simulink model "Control_v2"  (R2019b)
settings: Solver=FixedStepAuto  StartTime=0.0  StopTime=10  FixedStep=str2num(Step_size)  RelTol=1e-3
model workspace: external: MATLAB File H:\4-project\matlab\github\Sim-v2\bicopter_sim\Bicopter_DataFile14.m (data not in the file)
values from neighbouring files (symbols this model uses):
  b = [5,1,5,4]    [init_ADRC_val.m]    (also in init_Non_Linear_ADRC_val.m = 0.5*[1,    1, 6,  6]')
  b_sep = gains(5:8)    [get_ADRC_parameters.m]    (also in get_adrc_sep.m = [  2   7    6   7]; get_adrc_sep_kalman.m = [  2   2    6   7])
  C = [eye(4),zeros(4,8)]    [init_ADRC_val.m]
  C_air = 0.0025    [Sim_Script.m]
  d_f_phi = 100    [Sim_Script.m]
  d_f_psi = 25    [Sim_Script.m]
  d_f_theta = 10    [Sim_Script.m]
  d_f_z = 100    [Sim_Script.m]
  eps_sep = 0.7*[1 1 1 1]    [get_ADRC_parameters.m]    (also in get_adrc_sep.m = [0.7 0.3 0.3 0.35]; get_adrc_sep_kalman.m = [0.7 0.7 0.3 0.35])
  epsi = 1.5    [init_Non_Linear_ADRC_val.m]
  euler_source = 1    [Sim_Script.m]
  freq_cut_angvel_phi = 75    [Sim_Script.m]
  freq_cut_angvel_psi = 75    [Sim_Script.m]
  freq_cut_angvel_theta = 50    [Sim_Script.m]
  g = 9.81    [Sim_Script.m]
  K = place(A1,B1,w00(1:8))    [init_ADRC_val.m]
  L = place(A',C',8*w00)'    [init_ADRC_val.m]
  method = STSC_controller    (= 2)    [Sim_Script.m]
  method_angle_plane_sw = plane_sw    (= 2)    [Sim_Script.m]
  mult_obs = 10    [init_Non_Linear_ADRC_val.m]
  Noise_gain = 1    [Sim_Script.m]
  PID_VAL_SEP = init_pid_val_sep()    [Sim_Script.m]
  polarity = [-1;1;1;1]    [Sim_Script.m]
  r = [10,5,10,10]    [init_Non_Linear_ADRC_val.m]
  S_phi = 0.001    [Sim_Script.m]
  S_psi = S_phi    (= 0.001)    [Sim_Script.m]
  S_theta = S_phi    (= 0.001)    [Sim_Script.m]
  State_step = [Z_step;Phi_step;Theta_step;Psi_step]    [req_response.m]
  Step_size = step_size    [Sim_Script.m]
  STSC_VAL = init_STSC_val()    [Sim_Script.m]
  time_delay = 1e-6    (= 1e-06)    [Sim_Script.m]
  V_phi = 0.01    [Sim_Script.m]
  V_psi = 0.01    [Sim_Script.m]
  V_theta = 0.01    [Sim_Script.m]
  wc_sep = gains(1:4)    [get_ADRC_parameters.m]    (also in get_adrc_sep.m = [ 5.54   9   6    3]; get_adrc_sep_kalman.m = [ 5.54   9   6    3])
  wo_sep = ga*wc_sep    [get_ADRC_parameters.m]    (also in get_adrc_sep.m; get_adrc_sep_kalman.m)
undefined symbols (not defined in the file or in its folder): Continuous, magnitude, NLADRC_VAL, sigbuilder_block, smiData, Time, X, Y, Z
libraries: sm_lib x141, nesl_utility x20, simulink x19, fuzblock x3, sharedtransform x1, ctrlSharedLib x1
(part 7 of 7)

== system Control_v2/System/Controller/NonLinearADRC/controller_phi2/NLSEF/f_nl1 ==
  e : Inport
  Constant2 : Constant
  Divide : Product  Inputs=*/
  Power : Math  Operator=pow  SignedPower=off  SaturateOnIntegerOverflow=on
  Power1 : Math  Operator=pow  SignedPower=off  SaturateOnIntegerOverflow=on
  Product : Product
  Sign1 : Signum
  Subtract : Sum  Inputs=+-
  Switch : Switch  Criteria=u2 > Threshold  Threshold=NLADRC_VAL(ind,2)
  eta : Constant  Value=NLADRC_VAL(ind,2)
  gamma : Constant  Value=NLADRC_VAL(ind,3)
  fnl : Outport
  wires:
  Switch/1 -> fnl/1
  gamma/1 -> Subtract/1, Power/2
  [abs_err] -> Power/1
  Divide/1 -> Switch/3
  Power1/1 -> Divide/2
  Subtract/1 -> Power1/2
  eta/1 -> Power1/1
  [sign_err] -> Product/2
  Power/1 -> Product/1
  Constant2/1 -> Subtract/2
  e/1 -> [err], [abs_err], Sign1/1
  Product/1 -> Switch/1
  [abs_err] -> Switch/2
  Sign1/1 -> [sign_err]
  [err] -> Divide/1

== system Control_v2/System/Controller/NonLinearADRC/controller_phi3/NLSEF/f_nl ==
  e : Inport
  Constant2 : Constant
  Divide : Product  Inputs=*/
  Power : Math  Operator=pow  SignedPower=off  SaturateOnIntegerOverflow=on
  Power1 : Math  Operator=pow  SignedPower=off  SaturateOnIntegerOverflow=on
  Product : Product
  Sign1 : Signum
  Subtract : Sum  Inputs=+-
  Switch : Switch  Criteria=u2 > Threshold  Threshold=NLADRC_VAL(ind,2)
  eta : Constant  Value=NLADRC_VAL(ind,2)
  gamma : Constant  Value=NLADRC_VAL(ind,3)
  fnl : Outport
  wires:
  Switch/1 -> fnl/1
  gamma/1 -> Subtract/1, Power/2
  [abs_err] -> Power/1
  Divide/1 -> Switch/3
  Power1/1 -> Divide/2
  Subtract/1 -> Power1/2
  eta/1 -> Power1/1
  [sign_err] -> Product/2
  Power/1 -> Product/1
  Constant2/1 -> Subtract/2
  e/1 -> [err], [abs_err], Sign1/1
  Product/1 -> Switch/1
  [abs_err] -> Switch/2
  Sign1/1 -> [sign_err]
  [err] -> Divide/1

== system Control_v2/System/Controller/NonLinearADRC/controller_phi3/NLSEF/f_nl1 ==
  e : Inport
  Constant2 : Constant
  Divide : Product  Inputs=*/
  Power : Math  Operator=pow  SignedPower=off  SaturateOnIntegerOverflow=on
  Power1 : Math  Operator=pow  SignedPower=off  SaturateOnIntegerOverflow=on
  Product : Product
  Sign1 : Signum
  Subtract : Sum  Inputs=+-
  Switch : Switch  Criteria=u2 > Threshold  Threshold=NLADRC_VAL(ind,2)
  eta : Constant  Value=NLADRC_VAL(ind,2)
  gamma : Constant  Value=NLADRC_VAL(ind,3)
  fnl : Outport
  wires:
  [err] -> Divide/1
  Sign1/1 -> [sign_err]
  [abs_err] -> Switch/2
  Product/1 -> Switch/1
  e/1 -> Sign1/1, [abs_err], [err]
  Constant2/1 -> Subtract/2
  Power/1 -> Product/1
  [sign_err] -> Product/2
  eta/1 -> Power1/1
  Subtract/1 -> Power1/2
  Power1/1 -> Divide/2
  Divide/1 -> Switch/3
  [abs_err] -> Power/1
  gamma/1 -> Power/2, Subtract/1
  Switch/1 -> fnl/1

== system Control_v2/System/Controller/NonLinearADRC/controller_z/NLSEF/f_nl ==
  e : Inport
  Constant2 : Constant
  Divide : Product  Inputs=*/
  Power : Math  Operator=pow  SignedPower=off  SaturateOnIntegerOverflow=on
  Power1 : Math  Operator=pow  SignedPower=off  SaturateOnIntegerOverflow=on
  Product : Product
  Sign1 : Signum
  Subtract : Sum  Inputs=+-
  Switch : Switch  Criteria=u2 > Threshold  Threshold=NLADRC_VAL(ind,2)
  eta : Constant  Value=NLADRC_VAL(ind,2)
  gamma : Constant  Value=NLADRC_VAL(ind,3)
  fnl : Outport
  wires:
  Switch/1 -> fnl/1
  gamma/1 -> Subtract/1, Power/2
  [abs_err] -> Power/1
  Divide/1 -> Switch/3
  Power1/1 -> Divide/2
  Subtract/1 -> Power1/2
  eta/1 -> Power1/1
  [sign_err] -> Product/2
  Power/1 -> Product/1
  Constant2/1 -> Subtract/2
  e/1 -> [err], [abs_err], Sign1/1
  Product/1 -> Switch/1
  [abs_err] -> Switch/2
  Sign1/1 -> [sign_err]
  [err] -> Divide/1

== system Control_v2/System/Controller/NonLinearADRC/controller_z/NLSEF/f_nl1 ==
  e : Inport
  Constant2 : Constant
  Divide : Product  Inputs=*/
  Power : Math  Operator=pow  SignedPower=off  SaturateOnIntegerOverflow=on
  Power1 : Math  Operator=pow  SignedPower=off  SaturateOnIntegerOverflow=on
  Product : Product
  Sign1 : Signum
  Subtract : Sum  Inputs=+-
  Switch : Switch  Criteria=u2 > Threshold  Threshold=NLADRC_VAL(ind,2)
  eta : Constant  Value=NLADRC_VAL(ind,2)
  gamma : Constant  Value=NLADRC_VAL(ind,3)
  fnl : Outport
  wires:
  [err] -> Divide/1
  Sign1/1 -> [sign_err]
  [abs_err] -> Switch/2
  Product/1 -> Switch/1
  e/1 -> Sign1/1, [abs_err], [err]
  Constant2/1 -> Subtract/2
  Power/1 -> Product/1
  [sign_err] -> Product/2
  eta/1 -> Power1/1
  Subtract/1 -> Power1/2
  Power1/1 -> Divide/2
  Divide/1 -> Switch/3
  [abs_err] -> Power/1
  gamma/1 -> Power/2, Subtract/1
  Switch/1 -> fnl/1

== matlab function Control_v2/System/Delay/MATLAB Function ==
  data: u input; P output; Euler output; V output; W output
function [P,Euler,V,W] = fcn(u)
P = u(1:3);
Euler = u(4:6);
V = u(7:9);
W = u (10:12);

== matlab function Control_v2/System/Decoupling function ==
  data: u input; y output
function y = fcn(u)
    function z = satval(val,ub,lb)
        if val<lb
            z = lb;
        elseif val>ub
            z=ub;
        else
         z = val;
        end
    end
sat_ang = 0.4;
sat_power = 7;
%
u_sat = u;
u_sat(1) = satval(u(1),5,-5);
u_sat(2) = satval(u(2),12,0); %12
u_sat(3) = satval(u(3),5,-5);
u_sat(4) = satval(u(4),5,-5);
u = u_sat;

%
%% Bicopter :
f1=(u_sat(2)+u_sat(1))/2;
f2=(u_sat(2)-u_sat(1))/2;
if(abs(u_sat(1)+u_sat(2))<0.001)
   a1=0;
else
   a1=(u_sat(3)+u_sat(4))/(u_sat(1)+u_sat(2));
end
if(abs(u_sat(1)-u_sat(2))<0.001)
   a2=0;
else
   a2=(u_sat(3)-u_sat(4))/(u_sat(2)-u_sat(1));
end
     % saturation
f1 = satval(f1,sat_power,0);
f2 = satval(f2,sat_power,0);
a1 = satval(a1,sat_ang,-sat_ang);
a2 = satval(a2,sat_ang,-sat_ang);
y=[f1 f2 a1 a2]';

end

== matlab function Control_v2/System/Controller/NonLinearADRC/controller_z/TD/sat ==
  data: x1 input; v0 input; y output; x2 input
function y = fcn(x1,v0,x2)
tmp = x1-v0+x2;
delta  = 0.0025;
if abs(tmp)< delta
    y = tmp;
else
y = sign(tmp);
end

== matlab function Control_v2/System/angvel_2_euler/angvel_2_eulvel ==
  data: angvel input; eulvel output; eul input
function eulvel = fcn(angvel,eul)
%% Bicopter :
    if(length(eul)== 1)
        neweul = [0;0;0];
    else 
        neweul = eul;
    end
    % eul = [psi, theta, phi];
    psi = neweul(1);
    theta = neweul(2);
    phi = neweul(3);
    A = [1 0 -sin(theta);0 cos(phi) sin(phi)*cos(theta);0 -sin(phi) cos(phi)*cos(theta)];
    %[dphi;dtheta;dpsi] = inv([1 0 -sin(theta);0 cos(theta) sin(phi)*cos(theta);0 -sin(phi) cos(phi)*cos(theta)])*angvel;
    %if abs(det(A))<1e-8
        %A = eye(3);
    %end
    % angvel = [phi_dot,theta_dot,psi_dot]
    %deuler = A*angvel;
    deuler = A\angvel;
    eulvel = [deuler(3);deuler(2);deuler(1)];
end

== matlab function Control_v2/System/Controller/super_twisting_controller1/STSC_Phi2/MATLAB Function ==
  data: u input; y output
function y = fcn(u)
delta = 0.05;
y = u/delta;
if(y>1)
    y=1;
else
    if(y<-1)
        y=-1;
    end
end
end

== matlab function Control_v2/System/Controller/super_twisting_controller1/STSC_Phi2/MATLAB Function1 ==
  data: u input; y output; error input
function y = fcn(u,error)
delta = 1;

y = u/delta;
if(y>10)
    y=10;
else
    if(y<-10)
        y=-10;
    end
end

if (error<0.05 && error > 0)
    y=2*y;
else
    if(error<0)
        y= y/3;
    end
end
end

== matlab function Control_v2/System/Controller/ADRC_Kalman/Phi_loop/MATLAB Function ==
  data: u input; y output
function y = fcn(u)
if (length(u) ~= 1)
    y = [0;0;0];
else
y = [0;u;0];
end
